simulink model "DC_grid_Dynamic"  (R2025a)
settings: Solver=VariableStepAuto  StartTime=0.0  StopTime=10.0  RelTol=1e-3
undefined symbols (not defined in the file): DC, From_nodes, Load_busesDC, R_Loads_DC
settings Model: Creator=atomas  LastModifiedBy=atomas

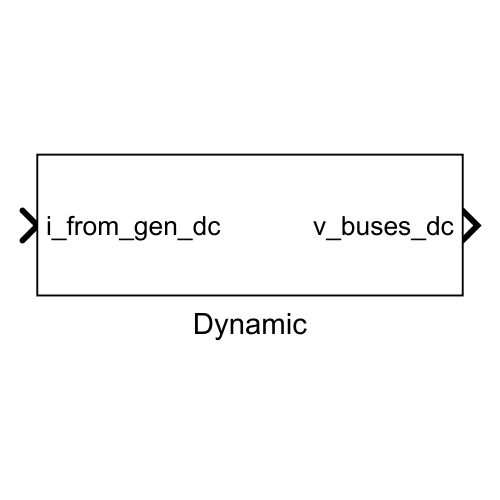
[thumbnail: Simulink's stored preview of the top-level diagram]
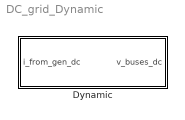
== system DC_grid_Dynamic ==
  Dynamic : Subsystem  VariantControl=Dynamic

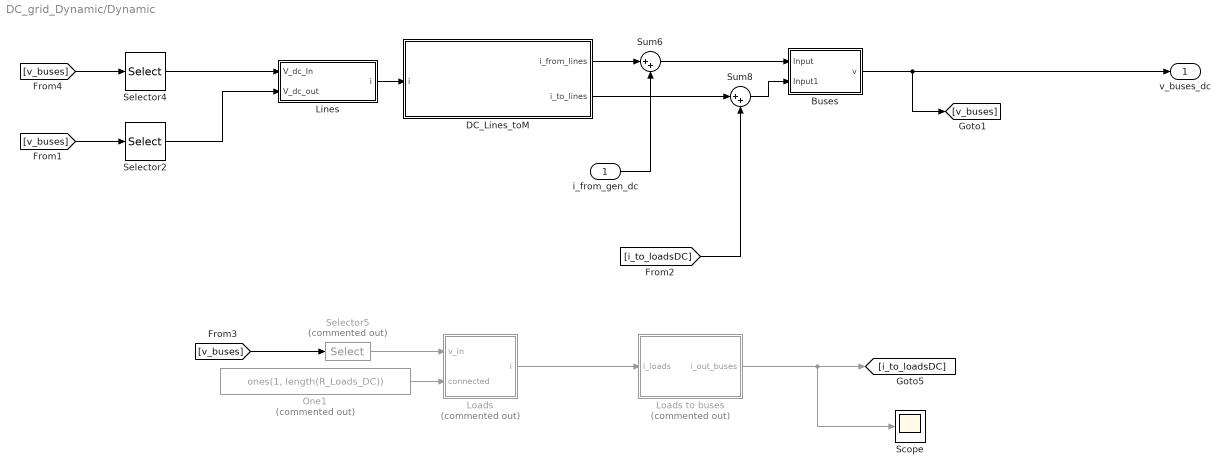
== system DC_grid_Dynamic/Dynamic ==
  i_from_gen_dc : Inport
  Buses : Subsystem
  DC_Lines_toM : Subsystem  TreatAsAtomicUnit=on
  Lines : Subsystem
  Loads : Subsystem  Commented=on
  Loads to buses : Subsystem  Commented=on
  One1 : Constant  Commented=on  Value=ones(1, length(R_Loads_DC))  VectorParams1D=off  OutDataTypeStr=Inherit: Inherit via back propagation
  Scope : Scope
      settings: ActiveDisplayYMinimum=-0.01246  ActiveDisplayYMaximum=0.11218
  Selector2 : Selector  NumberOfDimensions=2  InputPortWidth=Nnodes  IndexOptions=Select all,Index vector (dialog)  Indices=From_nodes,DC.to  OutputSizes=1,1
  Selector4 : Selector  NumberOfDimensions=2  InputPortWidth=Nnodes  IndexOptions=Select all,Index vector (dialog)  Indices=From_nodes,DC.from  OutputSizes=1,1
  Selector5 : Selector  Commented=on  NumberOfDimensions=2  InputPortWidth=Nnodes  IndexOptions=Select all,Index vector (dialog)  Indices=1,Load_busesDC  OutputSizes=1,1
  Sum6 : Sum  Inputs=|++
  Sum8 : Sum  Inputs=|++
  v_buses_dc : Outport
  wires:
  [v_buses] -> Selector5/1
  Loads to buses/1(i_out_buses) -> [i_to_loadsDC], Scope/1
  One1/1 -> Loads/2(connected)
  Lines/1(i) -> DC_Lines_toM/1(i)
  [i_to_loadsDC] -> Sum8/2
  [v_buses] -> Selector4/1
  DC_Lines_toM/1(i_from_lines) -> Sum6/1
  DC_Lines_toM/2(i_to_lines) -> Sum8/1
  Sum8/1 -> Buses/2(Input1)
  i_from_gen_dc/1 -> Sum6/2
  Selector5/1 -> Loads/1(v_in)
  Loads/1(i) -> Loads to buses/1(i_loads)
  Selector4/1 -> Lines/1(V_dc_In)
  Sum6/1 -> Buses/1(Input)
  Selector2/1 -> Lines/2(V_dc_out)
  [v_buses] -> Selector2/1
  Buses/1(v) -> [v_buses], v_buses_dc/1

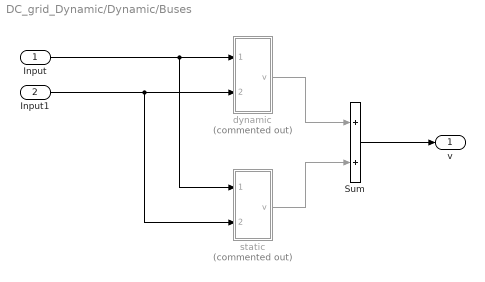
== system DC_grid_Dynamic/Dynamic/Buses ==
  Input : Inport
  Input1 : Inport  Port=2
  Sum : Sum
  dynamic : Subsystem  Commented=on
  static : Subsystem  Commented=on
  v : Outport
  wires:
  Sum/1 -> v/1
  static/1(v) -> Sum/2
  dynamic/1(v) -> Sum/1
  Input1/1 -> dynamic/2(i_out), static/2(i_out)
  Input/1 -> dynamic/1(i_in), static/1(i_in)

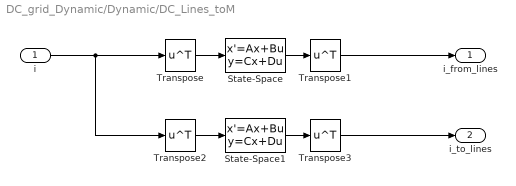
== system DC_grid_Dynamic/Dynamic/DC_Lines_toM ==
  i : Inport
  State-Space : StateSpace  A=[]  B=[]  C=[]  D=DC.Lines_toM  InitialCondition=0  ParameterTunability=Optimized
  State-Space1 : StateSpace  A=[]  B=[]  C=[]  D=DC.Lines_fromM  InitialCondition=0  ParameterTunability=Optimized
  Transpose{,1..3} (4 alike) : Math  Operator=transpose
  i_from_lines : Outport
  i_to_lines : Outport  Port=2
  wires:
  Transpose1/1 -> i_from_lines/1
  State-Space/1 -> Transpose1/1
  State-Space1/1 -> Transpose3/1
  Transpose/1 -> State-Space/1
  Transpose3/1 -> i_to_lines/1
  i/1 -> Transpose/1, Transpose2/1
  Transpose2/1 -> State-Space1/1

== system DC_grid_Dynamic/Dynamic/Lines ==
  V_dc_In : Inport
  V_dc_out : Inport  Port=2
  Dynamic : Subsystem  Commented=on
  Static : Subsystem  Commented=on
  Sum4 : Sum
  i : Outport
  wires:
  Sum4/1 -> i/1
  Static/1(i) -> Sum4/2
  Dynamic/1(i) -> Sum4/1
  V_dc_out/1 -> Static/2(V_dc_Out), Dynamic/2(V_dc_Out)
  V_dc_In/1 -> Dynamic/1(V_dc_In), Static/1(V_dc_In)

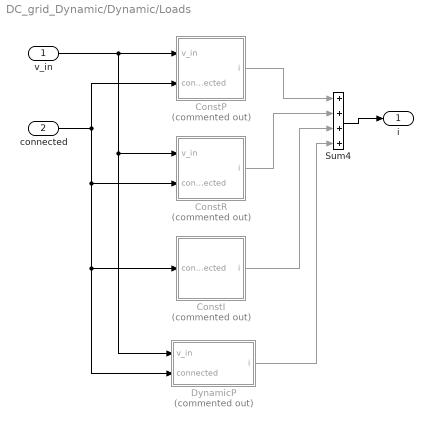
== system DC_grid_Dynamic/Dynamic/Loads ==
  v_in : Inport
  connected : Inport  Port=2
  ConstI : Subsystem  Commented=on
  ConstP : Subsystem  Commented=on
  ConstR : Subsystem  Commented=on
  DynamicP : Subsystem  Commented=on
  Sum4 : Sum  Inputs=++++
  i : Outport
  wires:
  DynamicP/1(i) -> Sum4/4
  ConstI/1(i) -> Sum4/3
  Sum4/1 -> i/1
  v_in/1 -> ConstP/1(v_in), ConstR/1(v_in), DynamicP/1(v_in)
  connected/1 -> ConstP/2(connected), ConstR/2(connected), ConstI/1(connected), DynamicP/2(connected)
  ConstP/1(i) -> Sum4/1
  ConstR/1(i) -> Sum4/2

== system DC_grid_Dynamic/Dynamic/Loads to buses ==
  i_loads : Inport
  LoadsM : Subsystem  TreatAsAtomicUnit=on
  i_out_buses : Outport
  wires:
  LoadsM/1(i_out_buses) -> i_out_buses/1
  i_loads/1 -> LoadsM/1(i)

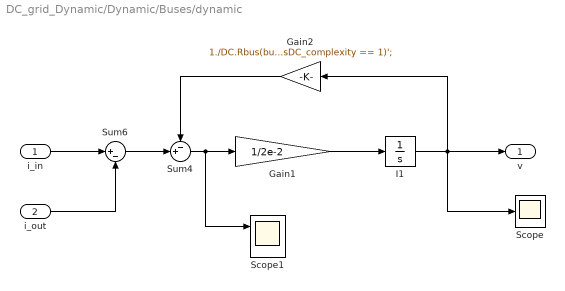
== system DC_grid_Dynamic/Dynamic/Buses/dynamic ==
  i_in : Inport
  i_out : Inport  Port=2
  Gain1 : Gain  Gain=1/2e-2
  Gain2 : Gain  Gain=1./DC.Rbus(busDC_complexity == 1)';
  I1 : Integrator  InitialCondition=DC.v(busDC_complexity == 1)
  Scope : Scope
      settings: ActiveDisplayYMinimum=0.9  ActiveDisplayYMaximum=1.1
  Scope1 : Scope  NumInputPorts=2
      settings: ActiveDisplayYMinimum=-0.35489510103335586  ActiveDisplayYMaximum=0.27003394850354928  DataLoggingVariableName=ScopeData5
  Sum4 : Sum  Inputs=-+|
  Sum6 : Sum  Inputs=|+-
  v : Outport
  wires:
  Gain1/1 -> I1/1
  i_out/1 -> Sum6/2
  Sum6/1 -> Sum4/2
  Sum4/1 -> Gain1/1, Scope1/1
  i_in/1 -> Sum6/1
  I1/1 -> Gain2/1, v/1, Scope/1
  Gain2/1 -> Sum4/1

== system DC_grid_Dynamic/Dynamic/Buses/static ==
  i_in : Inport
  i_out : Inport  Port=2
  Gain : Gain  Gain=1/1e-6
  LPF_d1 : Subsystem
  Sum1 : Sum  Inputs=+-
  v : Outport
  wires:
  LPF_d1/1(v_buses_dc) -> v/1
  Gain/1 -> LPF_d1/1(In1)
  i_out/1 -> Sum1/2
  i_in/1 -> Sum1/1
  Sum1/1 -> Gain/1

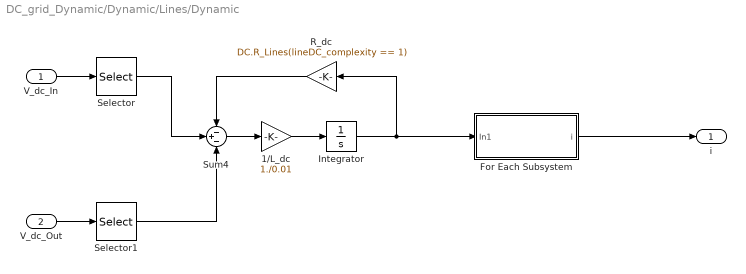
== system DC_grid_Dynamic/Dynamic/Lines/Dynamic ==
  V_dc_In : Inport
  V_dc_Out : Inport  Port=2
  1/L_dc : Gain  Gain=1./0.01
  For Each Subsystem : Subsystem  TreatAsAtomicUnit=on
  Integrator : Integrator  InitialCondition=DC.i_branch(lineDC_complexity == 1)
  R_dc : Gain  Gain=DC.R_Lines(lineDC_complexity == 1)
  Selector : Selector  NumberOfDimensions=2  InputPortWidth=3  IndexOptions=Index vector (dialog),Index vector (dialog)  Indices=1,find(lineDC_complexity == 1)  OutputSizes=1,1
  Selector1 : Selector  NumberOfDimensions=2  InputPortWidth=3  IndexOptions=Index vector (dialog),Index vector (dialog)  Indices=1,find(lineDC_complexity == 1)  OutputSizes=1,1
  Sum4 : Sum  Inputs=-+-
  i : Outport
  wires:
  Selector1/1 -> Sum4/3
  Selector/1 -> Sum4/2
  V_dc_In/1 -> Selector/1
  V_dc_Out/1 -> Selector1/1
  For Each Subsystem/1(i) -> i/1
  R_dc/1 -> Sum4/1
  1/L_dc/1 -> Integrator/1
  Sum4/1 -> 1/L_dc/1
  Integrator/1 -> R_dc/1, For Each Subsystem/1(In1)

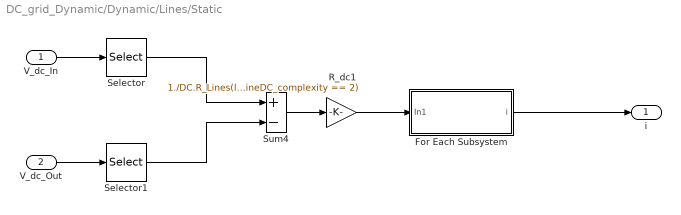
== system DC_grid_Dynamic/Dynamic/Lines/Static ==
  V_dc_In : Inport
  V_dc_Out : Inport  Port=2
  For Each Subsystem : Subsystem  TreatAsAtomicUnit=on
  R_dc1 : Gain  Gain=1./DC.R_Lines(lineDC_complexity == 2)
  Selector : Selector  NumberOfDimensions=2  InputPortWidth=3  IndexOptions=Index vector (dialog),Index vector (dialog)  Indices=1,find(lineDC_complexity == 2)  OutputSizes=1,1
  Selector1 : Selector  NumberOfDimensions=2  InputPortWidth=3  IndexOptions=Index vector (dialog),Index vector (dialog)  Indices=1,find(lineDC_complexity == 2)  OutputSizes=1,1
  Sum4 : Sum  Inputs=+-
  i : Outport
  wires:
  Selector1/1 -> Sum4/2
  V_dc_Out/1 -> Selector1/1
  Selector/1 -> Sum4/1
  V_dc_In/1 -> Selector/1
  For Each Subsystem/1(i) -> i/1
  R_dc1/1 -> For Each Subsystem/1(In1)
  Sum4/1 -> R_dc1/1

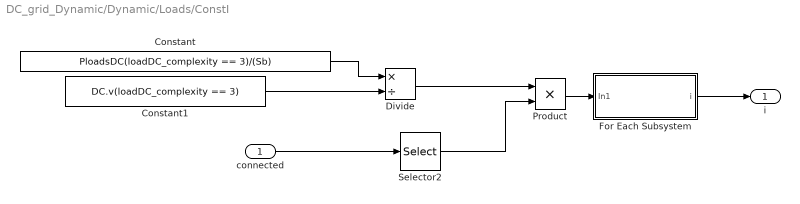
== system DC_grid_Dynamic/Dynamic/Loads/ConstI ==
  connected : Inport
  Constant : Constant  Value=PloadsDC(loadDC_complexity == 3)/(Sb)
  Constant1 : Constant  Value=DC.v(loadDC_complexity == 3)
  Divide : Product  Inputs=*/
  For Each Subsystem : Subsystem  TreatAsAtomicUnit=on
  Product : Product
  Selector2 : Selector  InputPortWidth=length(R_Loads_DC)  IndexOptions=Index vector (dialog)  Indices=find(loadDC_complexity == 3)  OutputSizes=1
  i : Outport
  wires:
  Divide/1 -> Product/1
  Constant1/1 -> Divide/2
  Constant/1 -> Divide/1
  For Each Subsystem/1(i) -> i/1
  Product/1 -> For Each Subsystem/1(In1)
  Selector2/1 -> Product/2
  connected/1 -> Selector2/1

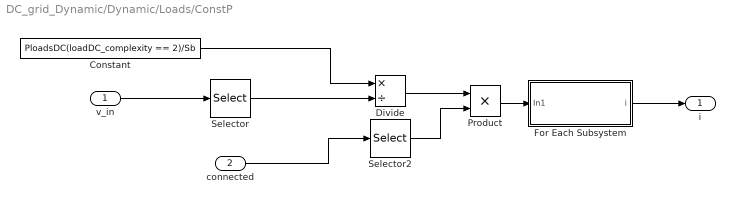
== system DC_grid_Dynamic/Dynamic/Loads/ConstP ==
  v_in : Inport
  connected : Inport  Port=2
  Constant : Constant  Value=PloadsDC(loadDC_complexity == 2)/Sb  VectorParams1D=off
  Divide : Product  Inputs=*/
  For Each Subsystem : Subsystem  TreatAsAtomicUnit=on
  Product : Product
  Selector : Selector  NumberOfDimensions=2  InputPortWidth=3  IndexOptions=Index vector (dialog),Index vector (dialog)  Indices=1,find(loadDC_complexity == 2)  OutputSizes=1,1
  Selector2 : Selector  InputPortWidth=length(R_Loads_DC)  IndexOptions=Index vector (dialog)  Indices=find(loadDC_complexity == 2)  OutputSizes=1
  i : Outport
  wires:
  For Each Subsystem/1(i) -> i/1
  Product/1 -> For Each Subsystem/1(In1)
  Selector/1 -> Divide/2
  v_in/1 -> Selector/1
  Selector2/1 -> Product/2
  connected/1 -> Selector2/1
  Divide/1 -> Product/1
  Constant/1 -> Divide/1

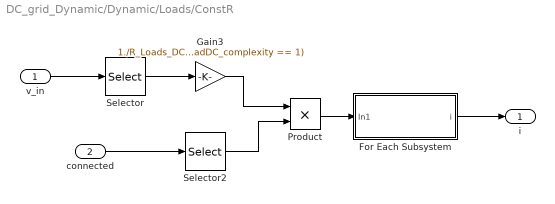
== system DC_grid_Dynamic/Dynamic/Loads/ConstR ==
  v_in : Inport
  connected : Inport  Port=2
  For Each Subsystem : Subsystem  TreatAsAtomicUnit=on
  Gain3 : Gain  Gain=1./R_Loads_DC(loadDC_complexity == 1)
  Product : Product
  Selector : Selector  NumberOfDimensions=2  InputPortWidth=3  IndexOptions=Index vector (dialog),Index vector (dialog)  Indices=1,find(loadDC_complexity == 1)  OutputSizes=1,1
  Selector2 : Selector  InputPortWidth=length(R_Loads_DC)  IndexOptions=Index vector (dialog)  Indices=find(loadDC_complexity == 1)  OutputSizes=1
  i : Outport
  wires:
  For Each Subsystem/1(i) -> i/1
  Product/1 -> For Each Subsystem/1(In1)
  Selector/1 -> Gain3/1
  v_in/1 -> Selector/1
  Selector2/1 -> Product/2
  connected/1 -> Selector2/1
  Gain3/1 -> Product/1

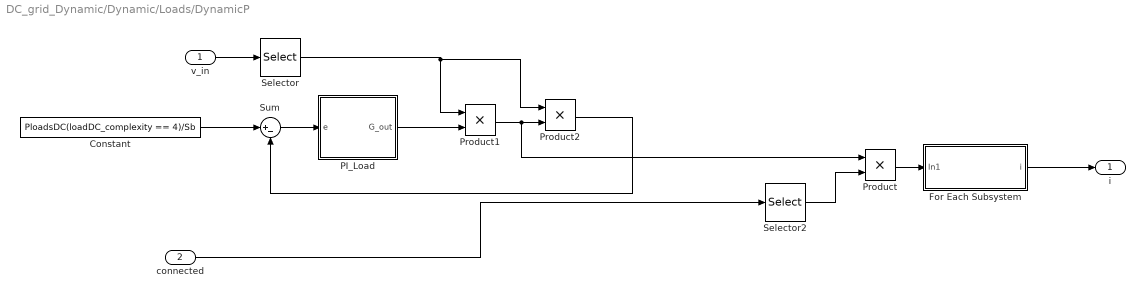
== system DC_grid_Dynamic/Dynamic/Loads/DynamicP ==
  v_in : Inport
  connected : Inport  Port=2
  Constant : Constant  Value=PloadsDC(loadDC_complexity == 4)/Sb
  For Each Subsystem : Subsystem  TreatAsAtomicUnit=on
  PI_Load : Subsystem
  Product : Product
  Product1 : Product
  Product2 : Product
  Selector : Selector  NumberOfDimensions=2  InputPortWidth=3  IndexOptions=Index vector (dialog),Index vector (dialog)  Indices=1,find(loadDC_complexity == 4)  OutputSizes=1,1
  Selector2 : Selector  InputPortWidth=length(R_Loads_DC)  IndexOptions=Index vector (dialog)  Indices=find(loadDC_complexity == 4)  OutputSizes=1
  Sum : Sum  Inputs=|+-
  i : Outport
  wires:
  Sum/1 -> PI_Load/1(e)
  PI_Load/1(G_out) -> Product1/2
  Product/1 -> For Each Subsystem/1(In1)
  For Each Subsystem/1(i) -> i/1
  Product1/1 -> Product2/2, Product/1
  Product2/1 -> Sum/2
  connected/1 -> Selector2/1
  Constant/1 -> Sum/1
  Selector2/1 -> Product/2
  v_in/1 -> Selector/1
  Selector/1 -> Product1/1, Product2/1

== system DC_grid_Dynamic/Dynamic/Loads to buses/LoadsM ==
  i : Inport  Partition=on  PartitionDimension=1  PartitionWidth=1  PartitionOffset=0
  Assignment : Assignment  DiagnosticForDimensions=Warning  IndexOptions=Index vector (dialog)  Indices=Load_busesDC  OutputSizes=1
  For Each : ForEach  DisableCoverage=on
  Zero : Constant  Value=zeros(1,DC.Nbuses)  VectorParams1D=off  OutDataTypeStr=Inherit: Inherit via back propagation
  i_out_buses : Outport  ConcatenationDimension=1
  wires:
  Zero/1 -> Assignment/1
  i/1 -> Assignment/2
  Assignment/1 -> i_out_buses/1

== system DC_grid_Dynamic/Dynamic/Buses/static/LPF_d1 ==
  In1 : Inport
  Gain : Gain  Gain=100
  I : Integrator  InitialCondition=DC.v(busDC_complexity == 2)
  Sum4 : Sum  Inputs=|+-
  v_buses_dc : Outport
  wires:
  I/1 -> Sum4/2, v_buses_dc/1
  In1/1 -> Sum4/1
  Sum4/1 -> Gain/1
  Gain/1 -> I/1

== system DC_grid_Dynamic/Dynamic/Lines/Dynamic/For Each Subsystem ==
  In1 : Inport  Partition=on  PartitionDimension=1  PartitionWidth=1  PartitionOffset=0
  Assignment : Assignment  DiagnosticForDimensions=Warning  IndexOptions=Index vector (dialog)  Indices=find(lineDC_complexity == 1)  OutputSizes=1
  For Each : ForEach  DisableCoverage=on
  Zero : Constant  Value=zeros(1,length(DC.from))  VectorParams1D=off  OutDataTypeStr=Inherit: Inherit via back propagation
  i : Outport  ConcatenationDimension=1
  wires:
  Zero/1 -> Assignment/1
  Assignment/1 -> i/1
  In1/1 -> Assignment/2

== system DC_grid_Dynamic/Dynamic/Lines/Static/For Each Subsystem ==
  In1 : Inport  Partition=on  PartitionDimension=1  PartitionWidth=1  PartitionOffset=0
  Assignment : Assignment  DiagnosticForDimensions=Warning  IndexOptions=Index vector (dialog)  Indices=find(lineDC_complexity == 2)  OutputSizes=1
  For Each : ForEach  DisableCoverage=on
  Zero : Constant  Value=zeros(1,length(DC.from))  VectorParams1D=off  OutDataTypeStr=Inherit: Inherit via back propagation
  i : Outport  ConcatenationDimension=1
  wires:
  Zero/1 -> Assignment/1
  Assignment/1 -> i/1
  In1/1 -> Assignment/2

== system DC_grid_Dynamic/Dynamic/Loads/ConstI/For Each Subsystem ==
  In1 : Inport  Partition=on  PartitionDimension=1  PartitionWidth=1  PartitionOffset=0
  Assignment : Assignment  DiagnosticForDimensions=Warning  IndexOptions=Index vector (dialog)  Indices=find(loadDC_complexity == 3)  OutputSizes=1
  For Each : ForEach  DisableCoverage=on
  Zero : Constant  Value=zeros(1,length(R_Loads_DC))  VectorParams1D=off  OutDataTypeStr=Inherit: Inherit via back propagation
  i : Outport  ConcatenationDimension=1
  wires:
  Zero/1 -> Assignment/1
  Assignment/1 -> i/1
  In1/1 -> Assignment/2

== system DC_grid_Dynamic/Dynamic/Loads/ConstP/For Each Subsystem ==
  In1 : Inport  Partition=on  PartitionDimension=1  PartitionWidth=1  PartitionOffset=0
  Assignment : Assignment  DiagnosticForDimensions=Warning  IndexOptions=Index vector (dialog)  Indices=find(loadDC_complexity == 2)  OutputSizes=1
  For Each : ForEach  DisableCoverage=on
  Zero : Constant  Value=zeros(1,length(R_Loads_DC))  VectorParams1D=off  OutDataTypeStr=Inherit: Inherit via back propagation
  i : Outport  ConcatenationDimension=1
  wires:
  Zero/1 -> Assignment/1
  Assignment/1 -> i/1
  In1/1 -> Assignment/2

== system DC_grid_Dynamic/Dynamic/Loads/ConstR/For Each Subsystem ==
  In1 : Inport  Partition=on  PartitionDimension=1  PartitionWidth=1  PartitionOffset=0
  Assignment : Assignment  DiagnosticForDimensions=Warning  IndexOptions=Index vector (dialog)  Indices=find(loadDC_complexity == 1)  OutputSizes=1
  For Each : ForEach  DisableCoverage=on
  Zero : Constant  Value=zeros(1,length(R_Loads_DC))  VectorParams1D=off  OutDataTypeStr=Inherit: Inherit via back propagation
  i : Outport  ConcatenationDimension=1
  wires:
  Zero/1 -> Assignment/1
  Assignment/1 -> i/1
  In1/1 -> Assignment/2

== system DC_grid_Dynamic/Dynamic/Loads/DynamicP/For Each Subsystem ==
  In1 : Inport  Partition=on  PartitionDimension=1  PartitionWidth=1  PartitionOffset=0
  Assignment : Assignment  DiagnosticForDimensions=Warning  IndexOptions=Index vector (dialog)  Indices=find(loadDC_complexity == 4)  OutputSizes=1
  For Each : ForEach  DisableCoverage=on
  Zero : Constant  Value=zeros(1,length(R_Loads_DC))  VectorParams1D=off  OutDataTypeStr=Inherit: Inherit via back propagation
  i : Outport  ConcatenationDimension=1
  wires:
  Zero/1 -> Assignment/1
  Assignment/1 -> i/1
  In1/1 -> Assignment/2

== system DC_grid_Dynamic/Dynamic/Loads/DynamicP/PI_Load ==
  e : Inport
  Gain : Gain  Gain=0.1/(100*pi)
  Gain1 : Gain  Gain=0.2/(100*pi)
  I : Integrator  InitialCondition=1./R_Loads_DC(loadDC_complexity == 4)
  Sum10 : Sum  Inputs=|++
  G_out : Outport
  wires:
  Sum10/1 -> G_out/1
  Gain/1 -> Sum10/1
  I/1 -> Sum10/2
  Gain1/1 -> I/1
  e/1 -> Gain/1, Gain1/1
